simulink model "ModemFM"  (R2020a)
settings: Solver=VariableStepAuto  StartTime=0.0  StopTime=1  MaxStep=1e-3  RelTol=1e-3
undefined symbols (not defined in the file or in its folder): Ap, Kf, wc, wm
settings Model: Creator=a1  LastModifiedBy=a1

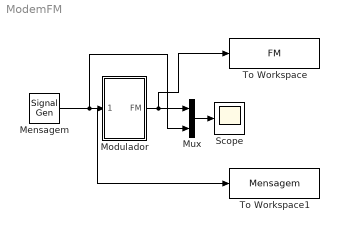
== system ModemFM ==
  " Mensagem" : SignalGenerator  Amplitude=Ap  Frequency=wm  Units=rad/sec
  Modulador : Subsystem
  Mux : Mux  Inputs=2
  Scope : Scope
  To Workspace : ToWorkspace  VariableName=FM  SampleTime=-1
  To Workspace1 : ToWorkspace  VariableName=Mensagem  SampleTime=-1
  wires:
  " Mensagem"/1 -> To Workspace1/1, Mux/2, Modulador/1(m(t))
  Modulador/1(FM) -> To Workspace/1, Mux/1
  Mux/1 -> Scope/1

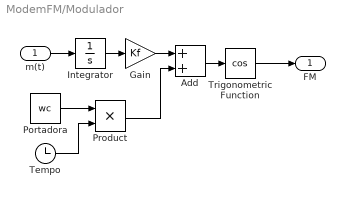
== system ModemFM/Modulador ==
  m(t) : Inport
  Add : Sum
  Gain : Gain  Gain=Kf
  Integrator : Integrator
  Portadora : Constant  Value=wc
  Product : Product
  Tempo : Clock
  Trigonometric Function : Trigonometry  Operator=cos
  FM : Outport
  wires:
  Tempo/1 -> Product/2
  Product/1 -> Add/2
  Integrator/1 -> Gain/1
  Trigonometric Function/1 -> FM/1
  Gain/1 -> Add/1
  m(t)/1 -> Integrator/1
  Add/1 -> Trigonometric Function/1
  Portadora/1 -> Product/1
